simulink model "LANDICHO_MACARAIG_NUMBER 2"  (R2024a)
settings: Solver=VariableStepAuto  StartTime=0.0  StopTime=20  RelTol=1e-3
values from neighbouring files (symbols this model uses):
  EQ10_den = conv(EQ10_den_cons, EQ9_num)    [LANDICHO_MACARAIG_NUMBER 2.m]
  EQ10_num = conv(EQ9_num, EQ10_num_cons)    [LANDICHO_MACARAIG_NUMBER 2.m]
  G1_den = [1 0 0]    [BERNABE_UNIGO_NUMBER1.m]    (also in LANDICHO_MACARAIG_NUMBER 2.m)
  G1_num = [1]    [BERNABE_UNIGO_NUMBER1.m]    (also in LANDICHO_MACARAIG_NUMBER 2.m = 1)
  G2_den = [1 1]    [BERNABE_UNIGO_NUMBER1.m]    (also in LANDICHO_MACARAIG_NUMBER 2.m)
  G2_num = [1]    [BERNABE_UNIGO_NUMBER1.m]    (also in LANDICHO_MACARAIG_NUMBER 2.m = 1)
  G3_den = [1 0]    [BERNABE_UNIGO_NUMBER1.m]    (also in LANDICHO_MACARAIG_NUMBER 2.m)
  G3_num = [1]    [BERNABE_UNIGO_NUMBER1.m]    (also in LANDICHO_MACARAIG_NUMBER 2.m = 1)
  G4_den = [2 0]    [LANDICHO_MACARAIG_NUMBER 2.m]
  G4_num = 1    [LANDICHO_MACARAIG_NUMBER 2.m]
  H1_den = [1 0]    [BERNABE_UNIGO_NUMBER1.m]    (also in LANDICHO_MACARAIG_NUMBER 2.m)
  H1_num = [1]    [BERNABE_UNIGO_NUMBER1.m]    (also in LANDICHO_MACARAIG_NUMBER 2.m = 1)
  H2_den = [1 -1]    [BERNABE_UNIGO_NUMBER1.m]    (also in LANDICHO_MACARAIG_NUMBER 2.m)
  H2_num = [1]    [BERNABE_UNIGO_NUMBER1.m]    (also in LANDICHO_MACARAIG_NUMBER 2.m = 1)
  H3_den = [1 -2]    [BERNABE_UNIGO_NUMBER1.m]    (also in LANDICHO_MACARAIG_NUMBER 2.m)
  H3_num = [1]    [BERNABE_UNIGO_NUMBER1.m]    (also in LANDICHO_MACARAIG_NUMBER 2.m = 1)

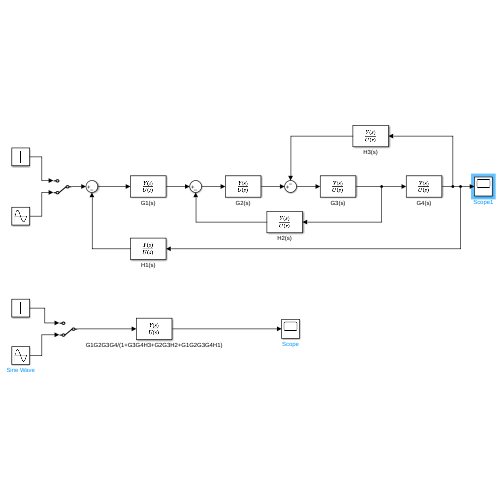
[thumbnail: Simulink's stored preview of the top-level diagram]
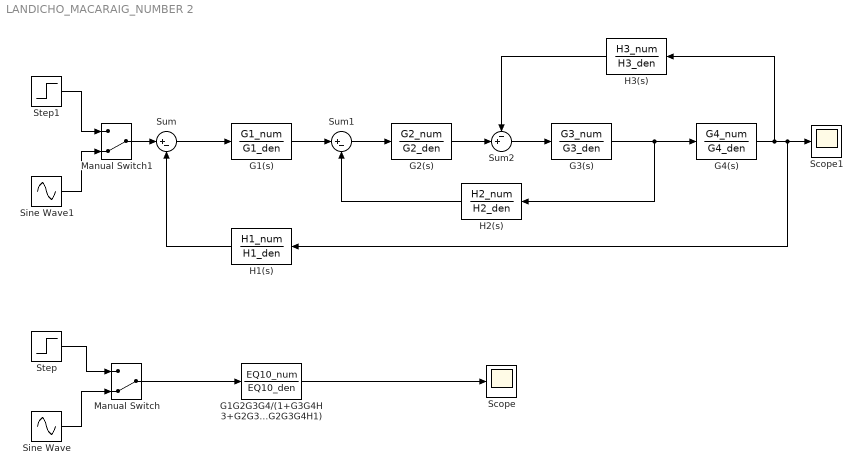
== system LANDICHO_MACARAIG_NUMBER 2 ==
  G1(s) : TransferFcn  Numerator=G1_num  Denominator=G1_den
  G1G2G3G4/(1+G3G4H3+G2G3H2+G1G2G3G4H1) : TransferFcn  Numerator=EQ10_num  Denominator=EQ10_den
  G2(s) : TransferFcn  Numerator=G2_num  Denominator=G2_den
  G3(s) : TransferFcn  Numerator=G3_num  Denominator=G3_den
  G4(s) : TransferFcn  Numerator=G4_num  Denominator=G4_den
  H1(s) : TransferFcn  Numerator=H1_num  Denominator=H1_den
  H2(s) : TransferFcn  Numerator=H2_num  Denominator=H2_den
  H3(s) : TransferFcn  Numerator=H3_num  Denominator=H3_den
  Manual Switch : ManualSwitch  CurrentSetting=0
  Manual Switch1 : ManualSwitch  CurrentSetting=0
  Scope : Scope
  Scope1 : Scope
  Sine Wave : Sin  SampleTime=0
  Sine Wave1 : Sin  SampleTime=0
  Step : Step  SampleTime=0
  Step1 : Step  Time=0  SampleTime=0
  Sum : Sum  Inputs=|+-
  Sum1 : Sum  Inputs=|+-
  Sum2 : Sum  Inputs=-+|
  wires:
  G1G2G3G4/(1+G3G4H3+G2G3H2+G1G2G3G4H1)/1 -> Scope/1
  Sine Wave/1 -> Manual Switch/2
  Manual Switch/1 -> G1G2G3G4/(1+G3G4H3+G2G3H2+G1G2G3G4H1)/1
  Step/1 -> Manual Switch/1
  Sine Wave1/1 -> Manual Switch1/2
  Step1/1 -> Manual Switch1/1
  G4(s)/1 -> H3(s)/1, H1(s)/1, Scope1/1
  G3(s)/1 -> H2(s)/1, G4(s)/1
  Manual Switch1/1 -> Sum/1
  Sum/1 -> G1(s)/1
  H1(s)/1 -> Sum/2
  G1(s)/1 -> Sum1/1
  H2(s)/1 -> Sum1/2
  Sum1/1 -> G2(s)/1
  G2(s)/1 -> Sum2/2
  Sum2/1 -> G3(s)/1
  H3(s)/1 -> Sum2/1
